simulink model "Robot"  (R2022b)
settings: Solver=FixedStepDiscrete  StartTime=0.0  StopTime=30  FixedStep=0.001  RelTol=1e-3
InitFcn:
  | load("BusConfig.mat");
undefined symbols (not defined in the file or in its folder): DiscIntNeverNeededParam
libraries: slrealtimeethercatlib x119, simulink x20
(part 1 of 7)
settings Model: SimulationMode=external  Creator=My-Dell-PC  LastModifiedBy=Lenovo
settings SolverCC: ConcurrentTasks=on  PositivePriorityOrder=on
settings OptimizationCC: BlockReduction=off  OptimizeBlockIOStorage=off
settings DebuggingCC: TasksWithSamePriorityMsg=none
settings HardwareCC: ProdBitPerLong=64  ProdLongLongMode=on  ProdHWDeviceType=Intel->x86-64 (Linux 64)
settings ModelReferenceCC: ModelReferenceNumInstancesAllowed=Single
settings RTWCC: Description=Simulink Real-Time  SystemTargetFile=slrealtime.tlc  TemplateMakefile=slrealtime_default_tmf  Toolchain=Simulink Real-Time Toolchain  BuildConfiguration=Faster Runs  CodeExecutionProfiling=on  TargetLang=C++
settings CodeAppCC: MaxIdLength=62

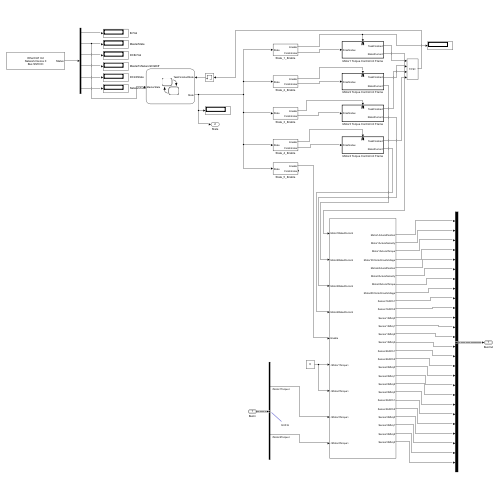
[thumbnail: Simulink's stored preview of the top-level diagram]
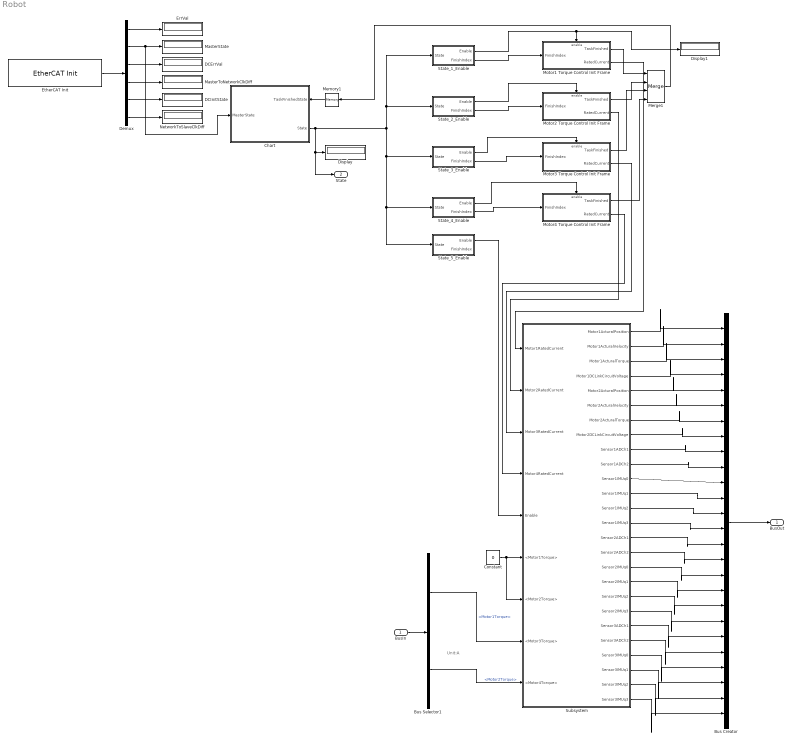
== system Robot ==
  note: Unit:A
  BusIn : Inport  OutDataTypeStr=Bus: ControlBus  BusOutputAsStruct=on
  Bus Creator : BusCreator  Inputs=26  OutDataTypeStr=Bus: SensingBus  NonVirtualBus=on
  Bus Selector1 : BusSelector  OutputSignals=Motor1Torque,Motor2Torque
  Chart : Stateflow chart  TreatAsAtomicUnit=on
      settings: PortSchema="{\"entries\":[{\"content\":{\"sides\":[{\"content\":{\"connectorIds\":[\"In2\"]},\"type\":\"ConnectorPlacement.EquallySpacedRectSide\",\"uuid\":\"7b8c9a1c-e183-4267-9de8-fd35f280369e\"},{\"content\":{\"connectorIds\":[\"In1\",\"Out1\"],\"side\":\"RIGHT\"},\"type\":\"ConnectorPlacement.EquallySpacedRectSide\",\"uuid\":\"78ba3a26-fd01-47d1-83ec-a88a58443a5d\"},{\"content\":{\"connectorIds\":[],\"side\":\"TOP\"},\"type\":\"ConnectorPlacement.EquallySpacedRectSide\",\"uuid\":\"d4867a2f-46dd-4a62-ab42-9e8e97143c91\"}]},\"type\":\"ConnectorPlacement.EquallySpacedConnector\",\"uuid\":\"fb86ace7-67ae-423a-b56c-83b1d93efbca\"}],\"packageUris\":[\"http://schema.mathworks.com/mf0/Connector/R2020b\"],\"version\":\"1.0\"}"
  Constant : Constant  Value=0
  "DCErrVal " : Display
  "DCInitState " : Display
  Demux : Demux  Outputs=6
  Display : Display
  Display1 : Display
  "ErrVal " : Display
  EtherCAT Init : slrealtimeethercatlib/EtherCAT Init  Priority=0  config_file=C:\Users\Lenovo\Desktop\Test03\FourMotorThreeSTMDevices.xml  device_id=0  pci_bus=0  pci_slot=0  pci_function=0  portnum=1  initstate=2  dctuning=0  enaDebug=1  enaDC=on  errLink=off  masterDbg=off  stateChgDbg=off  baseClock=off  masterCfg=off  logFile='c:\dbglog.txt'  sample_time=0.001000  DCMode=1
  "MasterState " : Display
  "MasterToNetworkClkDiff " : Display
  Memory1 : Memory
  Merge1 : Merge  Inputs=4
  Motor1 Torque Control Init Frame : Subsystem
  Motor2 Torque Control Init Frame : Subsystem
  Motor3 Torque Control Init Frame : Subsystem
  Motor4 Torque Control Init Frame : Subsystem
  "NetworkToSlaveClkDiff " : Display
  State_1_Enable : Subsystem  mask{TaskIndex=1}
  State_2_Enable : Subsystem  mask{TaskIndex=2}
  State_3_Enable : Subsystem  mask{TaskIndex=3}
  State_4_Enable : Subsystem  mask{TaskIndex=4}
  State_5_Enable : Subsystem  mask{TaskIndex=5}
  Subsystem : Subsystem
  BusOut : Outport  OutDataTypeStr=Bus: SensingBus  BusOutputAsStruct=on
  State : Outport  Port=2
  wires:
  Memory1/1 -> Chart/1(TaskFinishedState)
  State_1_Enable/2(FinishIndex) -> Motor1 Torque Control Init Frame/1(FinishIndex)
  Demux/1 -> "ErrVal "/1
  Merge1/1 -> Memory1/1
  Demux/6 -> "NetworkToSlaveClkDiff "/1
  Motor2 Torque Control Init Frame/1(TaskFinished) -> Merge1/2
  State_2_Enable/2(FinishIndex) -> Motor2 Torque Control Init Frame/1(FinishIndex)
  BusIn/1 -> Bus Selector1/1
  Motor1 Torque Control Init Frame/1(TaskFinished) -> Merge1/1
  Demux/4 -> "MasterToNetworkClkDiff "/1
  State_1_Enable/1(Enable) -> Motor1 Torque Control Init Frame/Enable, Display1/1
  State_2_Enable/1(Enable) -> Motor2 Torque Control Init Frame/Enable
  Demux/5 -> "DCInitState "/1
  EtherCAT Init/1 -> Demux/1
  Demux/2 -> "MasterState "/1, Chart/2(MasterState)
  Demux/3 -> "DCErrVal "/1
  Motor1 Torque Control Init Frame/2(RatedCurrent) -> Subsystem/1(Motor1RatedCurrent)
  Motor2 Torque Control Init Frame/2(RatedCurrent) -> Subsystem/2(Motor2RatedCurrent)
  State_5_Enable/1(Enable) -> Subsystem/5(Enable)
  Bus Selector1/1 -> Subsystem/8(<Motor3Torque>)  "<Motor1Torque>"
  Bus Selector1/2 -> Subsystem/9(<Motor4Torque>)  "<Motor2Torque>"
  Subsystem/1(Motor1ActuralPosition) -> Bus Creator/1
  Subsystem/2(Motor1ActuralVelocity) -> Bus Creator/2
  Subsystem/3(Motor1ActuralTorque) -> Bus Creator/3
  Subsystem/4(Motor1DCLinkCircuitVoltage) -> Bus Creator/4
  Subsystem/5(Motor2ActuralPosition) -> Bus Creator/5
  Subsystem/6(Motor2ActuralVelocity) -> Bus Creator/6
  Subsystem/7(Motor2ActuralTorque) -> Bus Creator/7
  Subsystem/8(Motor2DCLinkCircuitVoltage) -> Bus Creator/8
  Subsystem/9(Sensor1ADCh1) -> Bus Creator/9
  Subsystem/10(Sensor1ADCh2) -> Bus Creator/10
  Subsystem/11(Sensor1IMUq0) -> Bus Creator/11
  Subsystem/12(Sensor1IMUq1) -> Bus Creator/12
  Subsystem/13(Sensor1IMUq2) -> Bus Creator/13
  Subsystem/14(Sensor1IMUq3) -> Bus Creator/14
  Subsystem/15(Sensor2ADCh1) -> Bus Creator/15
  Subsystem/16(Sensor2ADCh2) -> Bus Creator/16
  Subsystem/17(Sensor2IMUq0) -> Bus Creator/17
  Subsystem/18(Sensor2IMUq1) -> Bus Creator/18
  Subsystem/19(Sensor2IMUq2) -> Bus Creator/19
  Subsystem/20(Sensor2IMUq3) -> Bus Creator/20
  Subsystem/21(Sensor3ADCh1) -> Bus Creator/21
  Subsystem/22(Sensor3ADCh2) -> Bus Creator/22
  Subsystem/23(Sensor3IMUq0) -> Bus Creator/23
  Subsystem/24(Sensor3IMUq1) -> Bus Creator/24
  Subsystem/25(Sensor3IMUq2) -> Bus Creator/25
  Subsystem/26(Sensor3IMUq3) -> Bus Creator/26
  Bus Creator/1 -> BusOut/1
  State_3_Enable/1(Enable) -> Motor3 Torque Control Init Frame/Enable
  State_3_Enable/2(FinishIndex) -> Motor3 Torque Control Init Frame/1(FinishIndex)
  Motor3 Torque Control Init Frame/1(TaskFinished) -> Merge1/3
  State_4_Enable/1(Enable) -> Motor4 Torque Control Init Frame/Enable
  State_4_Enable/2(FinishIndex) -> Motor4 Torque Control Init Frame/1(FinishIndex)
  Motor4 Torque Control Init Frame/1(TaskFinished) -> Merge1/4
  Motor3 Torque Control Init Frame/2(RatedCurrent) -> Subsystem/3(Motor3RatedCurrent)
  Motor4 Torque Control Init Frame/2(RatedCurrent) -> Subsystem/4(Motor4RatedCurrent)
  Constant/1 -> Subsystem/7(<Motor2Torque>), Subsystem/6(<Motor1Torque>)
  Chart/1(State) -> State_1_Enable/1(State), State_2_Enable/1(State), State_3_Enable/1(State), State_4_Enable/1(State), State_5_Enable/1(State), State/1, Display/1

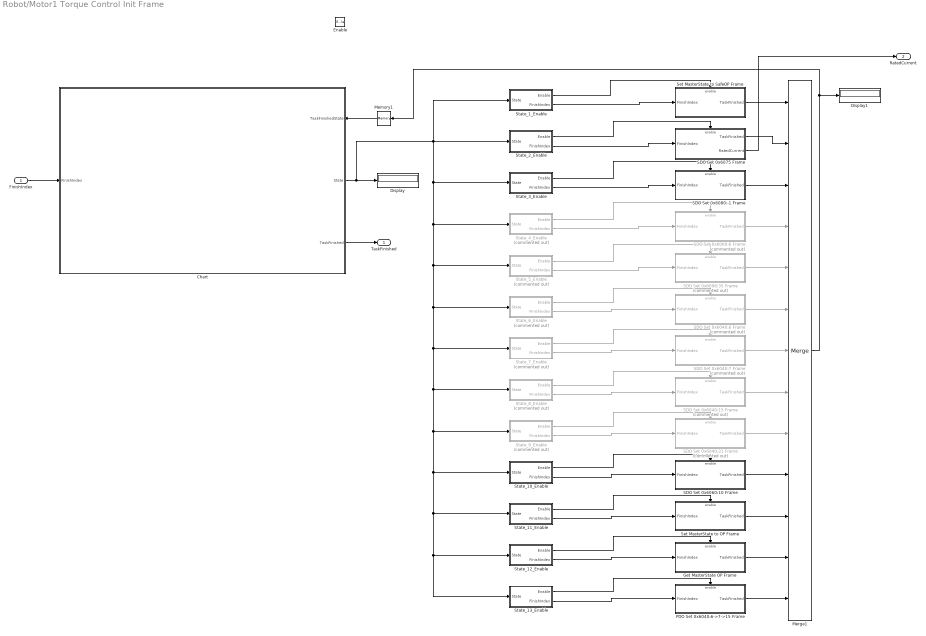
== system Robot/Motor1 Torque Control Init Frame ==
  FinishIndex : Inport
  Enable : EnablePort
  Chart : Stateflow chart  TreatAsAtomicUnit=on
      settings: PortSchema="{\"entries\":[{\"content\":{\"sides\":[{\"content\":{\"connectorIds\":[\"In1\"]},\"type\":\"ConnectorPlacement.EquallySpacedRectSide\",\"uuid\":\"58410e45-faf7-47e6-8ab9-12c4fba7eef9\"},{\"content\":{\"connectorIds\":[\"In2\",\"Out1\",\"Out2\"],\"side\":\"RIGHT\"},\"type\":\"ConnectorPlacement.EquallySpacedRectSide\",\"uuid\":\"b03d764f-4843-4a3f-88c0-0810c02290b2\"},{\"content\":{\"connectorIds\":[],\"side\":\"TOP\"},\"type\":\"ConnectorPlacement.EquallySpacedRectSide\",\"uuid\":\"d94600f9-94c4-4729-93e4-f24bdd83e939\"}]},\"type\":\"ConnectorPlacement.EquallySpacedConnector\",\"uuid\":\"f092a652-dcaf-4841-a284-968789b15227\"}],\"packageUris\":[\"http://schema.mathworks.com/mf0/Connector/R2020b\"],\"version\":\"1.0\"}"
  Display : Display
  Display1 : Display
  Get MasterState OP Frame : Subsystem
  Memory1 : Memory
  Merge1 : Merge  Inputs=13
  PDO Set 0x6040:6->7->15 Frame : Subsystem
  SDO Get 0x6075 Frame : Subsystem
  SDO Set 0x6040:15 Frame : Subsystem  Commented=on
  SDO Set 0x6040:31 Frame : Subsystem  Commented=on
  SDO Set 0x6040:6 Frame : Subsystem  Commented=on
  SDO Set 0x6040:7 Frame : Subsystem  Commented=on
  SDO Set 0x6060:10 Frame : Subsystem
  SDO Set 0x6060:6 Frame : Subsystem  Commented=on
  SDO Set 0x6080:-1 Frame : Subsystem
  SDO Set 0x6098:35 Frame : Subsystem  Commented=on
  Set MasterState to OP Frame : Subsystem
  Set MasterState to SafeOP Frame : Subsystem
  State_10_Enable : Subsystem  mask{TaskIndex=10}
  State_11_Enable : Subsystem  mask{TaskIndex=11}
  State_12_Enable : Subsystem  mask{TaskIndex=12}
  State_13_Enable : Subsystem  mask{TaskIndex=13}
  State_1_Enable : Subsystem  mask{TaskIndex=1}
  State_2_Enable : Subsystem  mask{TaskIndex=2}
  State_3_Enable : Subsystem  mask{TaskIndex=3}
  State_4_Enable : Subsystem  Commented=on  mask{TaskIndex=4}
  State_5_Enable : Subsystem  Commented=on  mask{TaskIndex=5}
  State_6_Enable : Subsystem  Commented=on  mask{TaskIndex=6}
  State_7_Enable : Subsystem  Commented=on  mask{TaskIndex=7}
  State_8_Enable : Subsystem  Commented=on  mask{TaskIndex=8}
  State_9_Enable : Subsystem  Commented=on  mask{TaskIndex=9}
  TaskFinished : Outport
  RatedCurrent : Outport  Port=2
  wires:
  SDO Get 0x6075 Frame/2(RatedCurrent) -> RatedCurrent/1
  Chart/1(State) -> State_1_Enable/1(State), State_2_Enable/1(State), State_3_Enable/1(State), State_4_Enable/1(State), State_5_Enable/1(State), State_6_Enable/1(State), State_7_Enable/1(State), State_8_Enable/1(State), State_9_Enable/1(State), State_10_Enable/1(State), State_11_Enable/1(State), State_13_Enable/1(State), State_12_Enable/1(State), Display/1
  Set MasterState to SafeOP Frame/1(TaskFinished) -> Merge1/1
  State_1_Enable/1(Enable) -> Set MasterState to SafeOP Frame/Enable
  State_1_Enable/2(FinishIndex) -> Set MasterState to SafeOP Frame/1(FinishIndex)
  State_2_Enable/1(Enable) -> SDO Get 0x6075 Frame/Enable
  State_2_Enable/2(FinishIndex) -> SDO Get 0x6075 Frame/1(FinishIndex)
  State_3_Enable/1(Enable) -> SDO Set 0x6080:-1 Frame/Enable
  State_3_Enable/2(FinishIndex) -> SDO Set 0x6080:-1 Frame/1(FinishIndex)
  State_4_Enable/1(Enable) -> SDO Set 0x6060:6 Frame/Enable
  State_4_Enable/2(FinishIndex) -> SDO Set 0x6060:6 Frame/1(FinishIndex)
  State_5_Enable/1(Enable) -> SDO Set 0x6098:35 Frame/Enable
  State_5_Enable/2(FinishIndex) -> SDO Set 0x6098:35 Frame/1(FinishIndex)
  State_6_Enable/1(Enable) -> SDO Set 0x6040:6 Frame/Enable
  State_6_Enable/2(FinishIndex) -> SDO Set 0x6040:6 Frame/1(FinishIndex)
  State_7_Enable/1(Enable) -> SDO Set 0x6040:7 Frame/Enable
  State_7_Enable/2(FinishIndex) -> SDO Set 0x6040:7 Frame/1(FinishIndex)
  State_8_Enable/2(FinishIndex) -> SDO Set 0x6040:15 Frame/1(FinishIndex)
  State_8_Enable/1(Enable) -> SDO Set 0x6040:15 Frame/Enable
  State_9_Enable/1(Enable) -> SDO Set 0x6040:31 Frame/Enable
  State_9_Enable/2(FinishIndex) -> SDO Set 0x6040:31 Frame/1(FinishIndex)
  State_10_Enable/1(Enable) -> SDO Set 0x6060:10 Frame/Enable
  State_10_Enable/2(FinishIndex) -> SDO Set 0x6060:10 Frame/1(FinishIndex)
  State_11_Enable/1(Enable) -> Set MasterState to OP Frame/Enable
  State_11_Enable/2(FinishIndex) -> Set MasterState to OP Frame/1(FinishIndex)
  State_12_Enable/1(Enable) -> Get MasterState OP Frame/Enable
  State_12_Enable/2(FinishIndex) -> Get MasterState OP Frame/1(FinishIndex)
  State_13_Enable/1(Enable) -> PDO Set 0x6040:6->7->15 Frame/Enable
  State_13_Enable/2(FinishIndex) -> PDO Set 0x6040:6->7->15 Frame/1(FinishIndex)
  SDO Get 0x6075 Frame/1(TaskFinished) -> Merge1/2
  SDO Set 0x6080:-1 Frame/1(TaskFinished) -> Merge1/3
  SDO Set 0x6060:6 Frame/1(TaskFinished) -> Merge1/4
  SDO Set 0x6098:35 Frame/1(TaskFinished) -> Merge1/5
  SDO Set 0x6040:6 Frame/1(TaskFinished) -> Merge1/6
  SDO Set 0x6040:7 Frame/1(TaskFinished) -> Merge1/7
  SDO Set 0x6040:15 Frame/1(TaskFinished) -> Merge1/8
  SDO Set 0x6040:31 Frame/1(TaskFinished) -> Merge1/9
  SDO Set 0x6060:10 Frame/1(TaskFinished) -> Merge1/10
  Set MasterState to OP Frame/1(TaskFinished) -> Merge1/11
  Get MasterState OP Frame/1(TaskFinished) -> Merge1/12
  PDO Set 0x6040:6->7->15 Frame/1(TaskFinished) -> Merge1/13
  Merge1/1 -> Display1/1, Memory1/1
  Chart/2(TaskFinished) -> TaskFinished/1
  FinishIndex/1 -> Chart/1(FinishIndex)
  Memory1/1 -> Chart/2(TaskFinishedState)

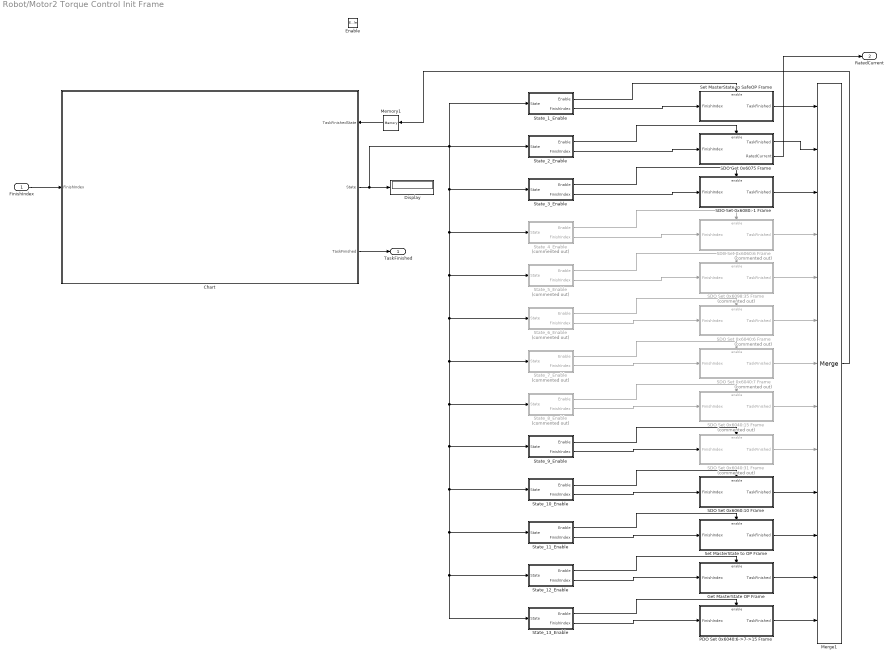
== system Robot/Motor2 Torque Control Init Frame ==
  FinishIndex : Inport
  Enable : EnablePort
  Chart : Stateflow chart  TreatAsAtomicUnit=on
      settings: PortSchema="{\"entries\":[{\"content\":{\"sides\":[{\"content\":{\"connectorIds\":[\"In1\"]},\"type\":\"ConnectorPlacement.EquallySpacedRectSide\",\"uuid\":\"58410e45-faf7-47e6-8ab9-12c4fba7eef9\"},{\"content\":{\"connectorIds\":[\"In2\",\"Out1\",\"Out2\"],\"side\":\"RIGHT\"},\"type\":\"ConnectorPlacement.EquallySpacedRectSide\",\"uuid\":\"b03d764f-4843-4a3f-88c0-0810c02290b2\"},{\"content\":{\"connectorIds\":[],\"side\":\"TOP\"},\"type\":\"ConnectorPlacement.EquallySpacedRectSide\",\"uuid\":\"d94600f9-94c4-4729-93e4-f24bdd83e939\"}]},\"type\":\"ConnectorPlacement.EquallySpacedConnector\",\"uuid\":\"f092a652-dcaf-4841-a284-968789b15227\"}],\"packageUris\":[\"http://schema.mathworks.com/mf0/Connector/R2020b\"],\"version\":\"1.0\"}"
  Display : Display
  Get MasterState OP Frame : Subsystem
  Memory1 : Memory
  Merge1 : Merge  Inputs=13
  PDO Set 0x6040:6->7->15 Frame : Subsystem
  SDO Get 0x6075 Frame : Subsystem
  SDO Set 0x6040:15 Frame : Subsystem  Commented=on
  SDO Set 0x6040:31 Frame : Subsystem  Commented=on
  SDO Set 0x6040:6 Frame : Subsystem  Commented=on
  SDO Set 0x6040:7 Frame : Subsystem  Commented=on
  SDO Set 0x6060:10 Frame : Subsystem
  SDO Set 0x6060:6 Frame : Subsystem  Commented=on
  SDO Set 0x6080:-1 Frame : Subsystem
  SDO Set 0x6098:35 Frame : Subsystem  Commented=on
  Set MasterState to OP Frame : Subsystem
  Set MasterState to SafeOP Frame : Subsystem
  State_10_Enable : Subsystem  mask{TaskIndex=10}
  State_11_Enable : Subsystem  mask{TaskIndex=11}
  State_12_Enable : Subsystem  mask{TaskIndex=12}
  State_13_Enable : Subsystem  mask{TaskIndex=13}
  State_1_Enable : Subsystem  mask{TaskIndex=1}
  State_2_Enable : Subsystem  mask{TaskIndex=2}
  State_3_Enable : Subsystem  mask{TaskIndex=3}
  State_4_Enable : Subsystem  Commented=on  mask{TaskIndex=4}
  State_5_Enable : Subsystem  Commented=on  mask{TaskIndex=5}
  State_6_Enable : Subsystem  Commented=on  mask{TaskIndex=6}
  State_7_Enable : Subsystem  Commented=on  mask{TaskIndex=7}
  State_8_Enable : Subsystem  Commented=on  mask{TaskIndex=8}
  State_9_Enable : Subsystem  mask{TaskIndex=9}
  TaskFinished : Outport
  RatedCurrent : Outport  Port=2
  wires:
  SDO Get 0x6075 Frame/2(RatedCurrent) -> RatedCurrent/1
  Chart/1(State) -> State_1_Enable/1(State), State_2_Enable/1(State), State_3_Enable/1(State), State_4_Enable/1(State), State_5_Enable/1(State), State_6_Enable/1(State), State_7_Enable/1(State), State_8_Enable/1(State), State_9_Enable/1(State), State_10_Enable/1(State), State_11_Enable/1(State), State_13_Enable/1(State), State_12_Enable/1(State), Display/1
  Set MasterState to SafeOP Frame/1(TaskFinished) -> Merge1/1
  State_1_Enable/1(Enable) -> Set MasterState to SafeOP Frame/Enable
  State_1_Enable/2(FinishIndex) -> Set MasterState to SafeOP Frame/1(FinishIndex)
  State_2_Enable/1(Enable) -> SDO Get 0x6075 Frame/Enable
  State_2_Enable/2(FinishIndex) -> SDO Get 0x6075 Frame/1(FinishIndex)
  State_3_Enable/1(Enable) -> SDO Set 0x6080:-1 Frame/Enable
  State_3_Enable/2(FinishIndex) -> SDO Set 0x6080:-1 Frame/1(FinishIndex)
  State_4_Enable/1(Enable) -> SDO Set 0x6060:6 Frame/Enable
  State_4_Enable/2(FinishIndex) -> SDO Set 0x6060:6 Frame/1(FinishIndex)
  State_5_Enable/1(Enable) -> SDO Set 0x6098:35 Frame/Enable
  State_5_Enable/2(FinishIndex) -> SDO Set 0x6098:35 Frame/1(FinishIndex)
  State_6_Enable/1(Enable) -> SDO Set 0x6040:6 Frame/Enable
  State_6_Enable/2(FinishIndex) -> SDO Set 0x6040:6 Frame/1(FinishIndex)
  State_7_Enable/1(Enable) -> SDO Set 0x6040:7 Frame/Enable
  State_7_Enable/2(FinishIndex) -> SDO Set 0x6040:7 Frame/1(FinishIndex)
  State_8_Enable/2(FinishIndex) -> SDO Set 0x6040:15 Frame/1(FinishIndex)
  State_8_Enable/1(Enable) -> SDO Set 0x6040:15 Frame/Enable
  State_9_Enable/1(Enable) -> SDO Set 0x6040:31 Frame/Enable
  State_9_Enable/2(FinishIndex) -> SDO Set 0x6040:31 Frame/1(FinishIndex)
  State_10_Enable/1(Enable) -> SDO Set 0x6060:10 Frame/Enable
  State_10_Enable/2(FinishIndex) -> SDO Set 0x6060:10 Frame/1(FinishIndex)
  State_11_Enable/1(Enable) -> Set MasterState to OP Frame/Enable
  State_11_Enable/2(FinishIndex) -> Set MasterState to OP Frame/1(FinishIndex)
  State_12_Enable/1(Enable) -> Get MasterState OP Frame/Enable
  State_12_Enable/2(FinishIndex) -> Get MasterState OP Frame/1(FinishIndex)
  State_13_Enable/1(Enable) -> PDO Set 0x6040:6->7->15 Frame/Enable
  State_13_Enable/2(FinishIndex) -> PDO Set 0x6040:6->7->15 Frame/1(FinishIndex)
  SDO Get 0x6075 Frame/1(TaskFinished) -> Merge1/2
  SDO Set 0x6080:-1 Frame/1(TaskFinished) -> Merge1/3
  SDO Set 0x6060:6 Frame/1(TaskFinished) -> Merge1/4
  SDO Set 0x6098:35 Frame/1(TaskFinished) -> Merge1/5
  SDO Set 0x6040:6 Frame/1(TaskFinished) -> Merge1/6
  SDO Set 0x6040:7 Frame/1(TaskFinished) -> Merge1/7
  SDO Set 0x6040:15 Frame/1(TaskFinished) -> Merge1/8
  SDO Set 0x6040:31 Frame/1(TaskFinished) -> Merge1/9
  SDO Set 0x6060:10 Frame/1(TaskFinished) -> Merge1/10
  Set MasterState to OP Frame/1(TaskFinished) -> Merge1/11
  Get MasterState OP Frame/1(TaskFinished) -> Merge1/12
  PDO Set 0x6040:6->7->15 Frame/1(TaskFinished) -> Merge1/13
  Merge1/1 -> Memory1/1
  Chart/2(TaskFinished) -> TaskFinished/1
  FinishIndex/1 -> Chart/1(FinishIndex)
  Memory1/1 -> Chart/2(TaskFinishedState)

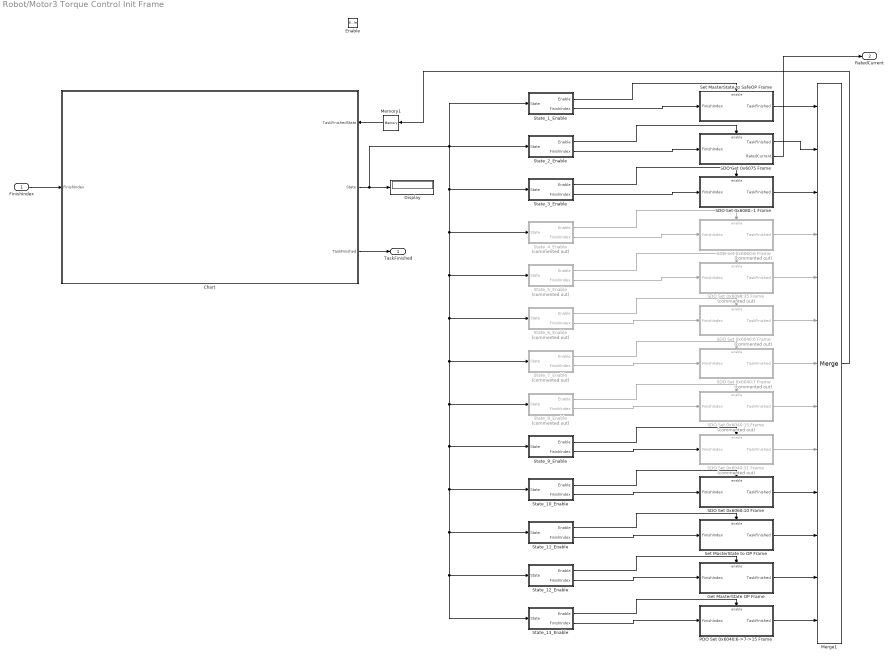
== system Robot/Motor3 Torque Control Init Frame ==
  FinishIndex : Inport
  Enable : EnablePort
  Chart : Stateflow chart  TreatAsAtomicUnit=on
      settings: PortSchema="{\"entries\":[{\"content\":{\"sides\":[{\"content\":{\"connectorIds\":[\"In1\"]},\"type\":\"ConnectorPlacement.EquallySpacedRectSide\",\"uuid\":\"58410e45-faf7-47e6-8ab9-12c4fba7eef9\"},{\"content\":{\"connectorIds\":[\"In2\",\"Out1\",\"Out2\"],\"side\":\"RIGHT\"},\"type\":\"ConnectorPlacement.EquallySpacedRectSide\",\"uuid\":\"b03d764f-4843-4a3f-88c0-0810c02290b2\"},{\"content\":{\"connectorIds\":[],\"side\":\"TOP\"},\"type\":\"ConnectorPlacement.EquallySpacedRectSide\",\"uuid\":\"d94600f9-94c4-4729-93e4-f24bdd83e939\"}]},\"type\":\"ConnectorPlacement.EquallySpacedConnector\",\"uuid\":\"f092a652-dcaf-4841-a284-968789b15227\"}],\"packageUris\":[\"http://schema.mathworks.com/mf0/Connector/R2020b\"],\"version\":\"1.0\"}"
  Display : Display
  Get MasterState OP Frame : Subsystem
  Memory1 : Memory
  Merge1 : Merge  Inputs=13
  PDO Set 0x6040:6->7->15 Frame : Subsystem
  SDO Get 0x6075 Frame : Subsystem
  SDO Set 0x6040:15 Frame : Subsystem  Commented=on
  SDO Set 0x6040:31 Frame : Subsystem  Commented=on
  SDO Set 0x6040:6 Frame : Subsystem  Commented=on
  SDO Set 0x6040:7 Frame : Subsystem  Commented=on
  SDO Set 0x6060:10 Frame : Subsystem
  SDO Set 0x6060:6 Frame : Subsystem  Commented=on
  SDO Set 0x6080:-1 Frame : Subsystem
  SDO Set 0x6098:35 Frame : Subsystem  Commented=on
  Set MasterState to OP Frame : Subsystem
  Set MasterState to SafeOP Frame : Subsystem
  State_10_Enable : Subsystem  mask{TaskIndex=10}
  State_11_Enable : Subsystem  mask{TaskIndex=11}
  State_12_Enable : Subsystem  mask{TaskIndex=12}
  State_13_Enable : Subsystem  mask{TaskIndex=13}
  State_1_Enable : Subsystem  mask{TaskIndex=1}
  State_2_Enable : Subsystem  mask{TaskIndex=2}
  State_3_Enable : Subsystem  mask{TaskIndex=3}
  State_4_Enable : Subsystem  Commented=on  mask{TaskIndex=4}
  State_5_Enable : Subsystem  Commented=on  mask{TaskIndex=5}
  State_6_Enable : Subsystem  Commented=on  mask{TaskIndex=6}
  State_7_Enable : Subsystem  Commented=on  mask{TaskIndex=7}
  State_8_Enable : Subsystem  Commented=on  mask{TaskIndex=8}
  State_9_Enable : Subsystem  mask{TaskIndex=9}
  TaskFinished : Outport
  RatedCurrent : Outport  Port=2
  wires:
  SDO Get 0x6075 Frame/2(RatedCurrent) -> RatedCurrent/1
  Chart/1(State) -> State_1_Enable/1(State), State_2_Enable/1(State), State_3_Enable/1(State), State_4_Enable/1(State), State_5_Enable/1(State), State_6_Enable/1(State), State_7_Enable/1(State), State_8_Enable/1(State), State_9_Enable/1(State), State_10_Enable/1(State), State_11_Enable/1(State), State_13_Enable/1(State), State_12_Enable/1(State), Display/1
  Set MasterState to SafeOP Frame/1(TaskFinished) -> Merge1/1
  State_1_Enable/1(Enable) -> Set MasterState to SafeOP Frame/Enable
  State_1_Enable/2(FinishIndex) -> Set MasterState to SafeOP Frame/1(FinishIndex)
  State_2_Enable/1(Enable) -> SDO Get 0x6075 Frame/Enable
  State_2_Enable/2(FinishIndex) -> SDO Get 0x6075 Frame/1(FinishIndex)
  State_3_Enable/1(Enable) -> SDO Set 0x6080:-1 Frame/Enable
  State_3_Enable/2(FinishIndex) -> SDO Set 0x6080:-1 Frame/1(FinishIndex)
  State_4_Enable/1(Enable) -> SDO Set 0x6060:6 Frame/Enable
  State_4_Enable/2(FinishIndex) -> SDO Set 0x6060:6 Frame/1(FinishIndex)
  State_5_Enable/1(Enable) -> SDO Set 0x6098:35 Frame/Enable
  State_5_Enable/2(FinishIndex) -> SDO Set 0x6098:35 Frame/1(FinishIndex)
  State_6_Enable/1(Enable) -> SDO Set 0x6040:6 Frame/Enable
  State_6_Enable/2(FinishIndex) -> SDO Set 0x6040:6 Frame/1(FinishIndex)
  State_7_Enable/1(Enable) -> SDO Set 0x6040:7 Frame/Enable
  State_7_Enable/2(FinishIndex) -> SDO Set 0x6040:7 Frame/1(FinishIndex)
  State_8_Enable/2(FinishIndex) -> SDO Set 0x6040:15 Frame/1(FinishIndex)
  State_8_Enable/1(Enable) -> SDO Set 0x6040:15 Frame/Enable
  State_9_Enable/1(Enable) -> SDO Set 0x6040:31 Frame/Enable
  State_9_Enable/2(FinishIndex) -> SDO Set 0x6040:31 Frame/1(FinishIndex)
  State_10_Enable/1(Enable) -> SDO Set 0x6060:10 Frame/Enable
  State_10_Enable/2(FinishIndex) -> SDO Set 0x6060:10 Frame/1(FinishIndex)
  State_11_Enable/1(Enable) -> Set MasterState to OP Frame/Enable
  State_11_Enable/2(FinishIndex) -> Set MasterState to OP Frame/1(FinishIndex)
  State_12_Enable/1(Enable) -> Get MasterState OP Frame/Enable
  State_12_Enable/2(FinishIndex) -> Get MasterState OP Frame/1(FinishIndex)
  State_13_Enable/1(Enable) -> PDO Set 0x6040:6->7->15 Frame/Enable
  State_13_Enable/2(FinishIndex) -> PDO Set 0x6040:6->7->15 Frame/1(FinishIndex)
  SDO Get 0x6075 Frame/1(TaskFinished) -> Merge1/2
  SDO Set 0x6080:-1 Frame/1(TaskFinished) -> Merge1/3
  SDO Set 0x6060:6 Frame/1(TaskFinished) -> Merge1/4
  SDO Set 0x6098:35 Frame/1(TaskFinished) -> Merge1/5
  SDO Set 0x6040:6 Frame/1(TaskFinished) -> Merge1/6
  SDO Set 0x6040:7 Frame/1(TaskFinished) -> Merge1/7
  SDO Set 0x6040:15 Frame/1(TaskFinished) -> Merge1/8
  SDO Set 0x6040:31 Frame/1(TaskFinished) -> Merge1/9
  SDO Set 0x6060:10 Frame/1(TaskFinished) -> Merge1/10
  Set MasterState to OP Frame/1(TaskFinished) -> Merge1/11
  Get MasterState OP Frame/1(TaskFinished) -> Merge1/12
  PDO Set 0x6040:6->7->15 Frame/1(TaskFinished) -> Merge1/13
  Merge1/1 -> Memory1/1
  Chart/2(TaskFinished) -> TaskFinished/1
  FinishIndex/1 -> Chart/1(FinishIndex)
  Memory1/1 -> Chart/2(TaskFinishedState)

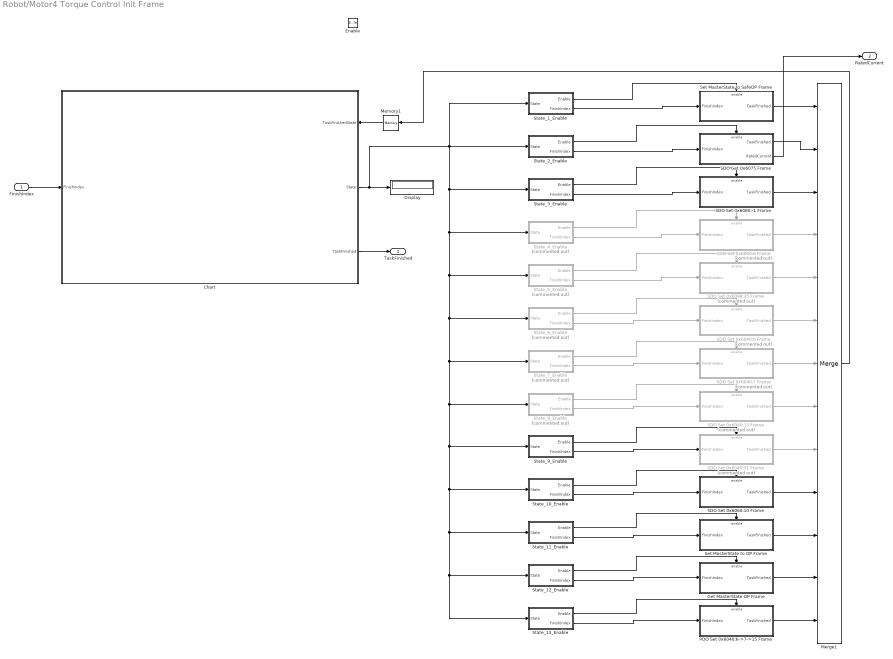
== system Robot/Motor4 Torque Control Init Frame ==
  FinishIndex : Inport
  Enable : EnablePort
  Chart : Stateflow chart  TreatAsAtomicUnit=on
      settings: PortSchema="{\"entries\":[{\"content\":{\"sides\":[{\"content\":{\"connectorIds\":[\"In1\"]},\"type\":\"ConnectorPlacement.EquallySpacedRectSide\",\"uuid\":\"58410e45-faf7-47e6-8ab9-12c4fba7eef9\"},{\"content\":{\"connectorIds\":[\"In2\",\"Out1\",\"Out2\"],\"side\":\"RIGHT\"},\"type\":\"ConnectorPlacement.EquallySpacedRectSide\",\"uuid\":\"b03d764f-4843-4a3f-88c0-0810c02290b2\"},{\"content\":{\"connectorIds\":[],\"side\":\"TOP\"},\"type\":\"ConnectorPlacement.EquallySpacedRectSide\",\"uuid\":\"d94600f9-94c4-4729-93e4-f24bdd83e939\"}]},\"type\":\"ConnectorPlacement.EquallySpacedConnector\",\"uuid\":\"f092a652-dcaf-4841-a284-968789b15227\"}],\"packageUris\":[\"http://schema.mathworks.com/mf0/Connector/R2020b\"],\"version\":\"1.0\"}"
  Display : Display
  Get MasterState OP Frame : Subsystem
  Memory1 : Memory
  Merge1 : Merge  Inputs=13
  PDO Set 0x6040:6->7->15 Frame : Subsystem
  SDO Get 0x6075 Frame : Subsystem
  SDO Set 0x6040:15 Frame : Subsystem  Commented=on
  SDO Set 0x6040:31 Frame : Subsystem  Commented=on
  SDO Set 0x6040:6 Frame : Subsystem  Commented=on
  SDO Set 0x6040:7 Frame : Subsystem  Commented=on
  SDO Set 0x6060:10 Frame : Subsystem
  SDO Set 0x6060:6 Frame : Subsystem  Commented=on
  SDO Set 0x6080:-1 Frame : Subsystem
  SDO Set 0x6098:35 Frame : Subsystem  Commented=on
  Set MasterState to OP Frame : Subsystem
  Set MasterState to SafeOP Frame : Subsystem
  State_10_Enable : Subsystem  mask{TaskIndex=10}
  State_11_Enable : Subsystem  mask{TaskIndex=11}
  State_12_Enable : Subsystem  mask{TaskIndex=12}
  State_13_Enable : Subsystem  mask{TaskIndex=13}
  State_1_Enable : Subsystem  mask{TaskIndex=1}
  State_2_Enable : Subsystem  mask{TaskIndex=2}
  State_3_Enable : Subsystem  mask{TaskIndex=3}
  State_4_Enable : Subsystem  Commented=on  mask{TaskIndex=4}
  State_5_Enable : Subsystem  Commented=on  mask{TaskIndex=5}
  State_6_Enable : Subsystem  Commented=on  mask{TaskIndex=6}
  State_7_Enable : Subsystem  Commented=on  mask{TaskIndex=7}
  State_8_Enable : Subsystem  Commented=on  mask{TaskIndex=8}
  State_9_Enable : Subsystem  mask{TaskIndex=9}
  TaskFinished : Outport
  RatedCurrent : Outport  Port=2
  wires:
  SDO Get 0x6075 Frame/2(RatedCurrent) -> RatedCurrent/1
  Chart/1(State) -> State_1_Enable/1(State), State_2_Enable/1(State), State_3_Enable/1(State), State_4_Enable/1(State), State_5_Enable/1(State), State_6_Enable/1(State), State_7_Enable/1(State), State_8_Enable/1(State), State_9_Enable/1(State), State_10_Enable/1(State), State_11_Enable/1(State), State_13_Enable/1(State), State_12_Enable/1(State), Display/1
  Set MasterState to SafeOP Frame/1(TaskFinished) -> Merge1/1
  State_1_Enable/1(Enable) -> Set MasterState to SafeOP Frame/Enable
  State_1_Enable/2(FinishIndex) -> Set MasterState to SafeOP Frame/1(FinishIndex)
  State_2_Enable/1(Enable) -> SDO Get 0x6075 Frame/Enable
  State_2_Enable/2(FinishIndex) -> SDO Get 0x6075 Frame/1(FinishIndex)
  State_3_Enable/1(Enable) -> SDO Set 0x6080:-1 Frame/Enable
  State_3_Enable/2(FinishIndex) -> SDO Set 0x6080:-1 Frame/1(FinishIndex)
  State_4_Enable/1(Enable) -> SDO Set 0x6060:6 Frame/Enable
  State_4_Enable/2(FinishIndex) -> SDO Set 0x6060:6 Frame/1(FinishIndex)
  State_5_Enable/1(Enable) -> SDO Set 0x6098:35 Frame/Enable
  State_5_Enable/2(FinishIndex) -> SDO Set 0x6098:35 Frame/1(FinishIndex)
  State_6_Enable/1(Enable) -> SDO Set 0x6040:6 Frame/Enable
  State_6_Enable/2(FinishIndex) -> SDO Set 0x6040:6 Frame/1(FinishIndex)
  State_7_Enable/1(Enable) -> SDO Set 0x6040:7 Frame/Enable
  State_7_Enable/2(FinishIndex) -> SDO Set 0x6040:7 Frame/1(FinishIndex)
  State_8_Enable/2(FinishIndex) -> SDO Set 0x6040:15 Frame/1(FinishIndex)
  State_8_Enable/1(Enable) -> SDO Set 0x6040:15 Frame/Enable
  State_9_Enable/1(Enable) -> SDO Set 0x6040:31 Frame/Enable
  State_9_Enable/2(FinishIndex) -> SDO Set 0x6040:31 Frame/1(FinishIndex)
  State_10_Enable/1(Enable) -> SDO Set 0x6060:10 Frame/Enable
  State_10_Enable/2(FinishIndex) -> SDO Set 0x6060:10 Frame/1(FinishIndex)
  State_11_Enable/1(Enable) -> Set MasterState to OP Frame/Enable
  State_11_Enable/2(FinishIndex) -> Set MasterState to OP Frame/1(FinishIndex)
  State_12_Enable/1(Enable) -> Get MasterState OP Frame/Enable
  State_12_Enable/2(FinishIndex) -> Get MasterState OP Frame/1(FinishIndex)
  State_13_Enable/1(Enable) -> PDO Set 0x6040:6->7->15 Frame/Enable
  State_13_Enable/2(FinishIndex) -> PDO Set 0x6040:6->7->15 Frame/1(FinishIndex)
  SDO Get 0x6075 Frame/1(TaskFinished) -> Merge1/2
  SDO Set 0x6080:-1 Frame/1(TaskFinished) -> Merge1/3
  SDO Set 0x6060:6 Frame/1(TaskFinished) -> Merge1/4
  SDO Set 0x6098:35 Frame/1(TaskFinished) -> Merge1/5
  SDO Set 0x6040:6 Frame/1(TaskFinished) -> Merge1/6
  SDO Set 0x6040:7 Frame/1(TaskFinished) -> Merge1/7
  SDO Set 0x6040:15 Frame/1(TaskFinished) -> Merge1/8
  SDO Set 0x6040:31 Frame/1(TaskFinished) -> Merge1/9
  SDO Set 0x6060:10 Frame/1(TaskFinished) -> Merge1/10
  Set MasterState to OP Frame/1(TaskFinished) -> Merge1/11
  Get MasterState OP Frame/1(TaskFinished) -> Merge1/12
  PDO Set 0x6040:6->7->15 Frame/1(TaskFinished) -> Merge1/13
  Merge1/1 -> Memory1/1
  Chart/2(TaskFinished) -> TaskFinished/1
  FinishIndex/1 -> Chart/1(FinishIndex)
  Memory1/1 -> Chart/2(TaskFinishedState)

== system Robot/State_1_Enable ==
  State : Inport
  Subsystem : Subsystem
  Switch Case : SwitchCase  CaseConditions={TaskIndex}
  Enable : Outport
  FinishIndex : Outport  Port=2
  wires:
  Switch Case/2 -> Subsystem/2(Case Default)
  Switch Case/1 -> Subsystem/1(Case)
  Subsystem/2(FinishIndex) -> FinishIndex/1
  Subsystem/1(Enable) -> Enable/1
  State/1 -> Switch Case/1

== system Robot/State_2_Enable ==
  State : Inport
  Subsystem : Subsystem
  Switch Case : SwitchCase  CaseConditions={TaskIndex}
  Enable : Outport
  FinishIndex : Outport  Port=2
  wires:
  Switch Case/2 -> Subsystem/2(Case Default)
  Switch Case/1 -> Subsystem/1(Case)
  Subsystem/2(FinishIndex) -> FinishIndex/1
  Subsystem/1(Enable) -> Enable/1
  State/1 -> Switch Case/1

== system Robot/State_3_Enable ==
  State : Inport
  Subsystem : Subsystem
  Switch Case : SwitchCase  CaseConditions={TaskIndex}
  Enable : Outport
  FinishIndex : Outport  Port=2
  wires:
  Switch Case/2 -> Subsystem/2(Case Default)
  Switch Case/1 -> Subsystem/1(Case)
  Subsystem/2(FinishIndex) -> FinishIndex/1
  Subsystem/1(Enable) -> Enable/1
  State/1 -> Switch Case/1

== system Robot/State_4_Enable ==
  State : Inport
  Subsystem : Subsystem
  Switch Case : SwitchCase  CaseConditions={TaskIndex}
  Enable : Outport
  FinishIndex : Outport  Port=2
  wires:
  Switch Case/2 -> Subsystem/2(Case Default)
  Switch Case/1 -> Subsystem/1(Case)
  Subsystem/2(FinishIndex) -> FinishIndex/1
  Subsystem/1(Enable) -> Enable/1
  State/1 -> Switch Case/1

== system Robot/State_5_Enable ==
  State : Inport
  Subsystem : Subsystem
  Switch Case : SwitchCase  CaseConditions={TaskIndex}
  Enable : Outport
  FinishIndex : Outport  Port=2
  wires:
  Switch Case/2 -> Subsystem/2(Case Default)
  Switch Case/1 -> Subsystem/1(Case)
  Subsystem/2(FinishIndex) -> FinishIndex/1
  Subsystem/1(Enable) -> Enable/1
  State/1 -> Switch Case/1

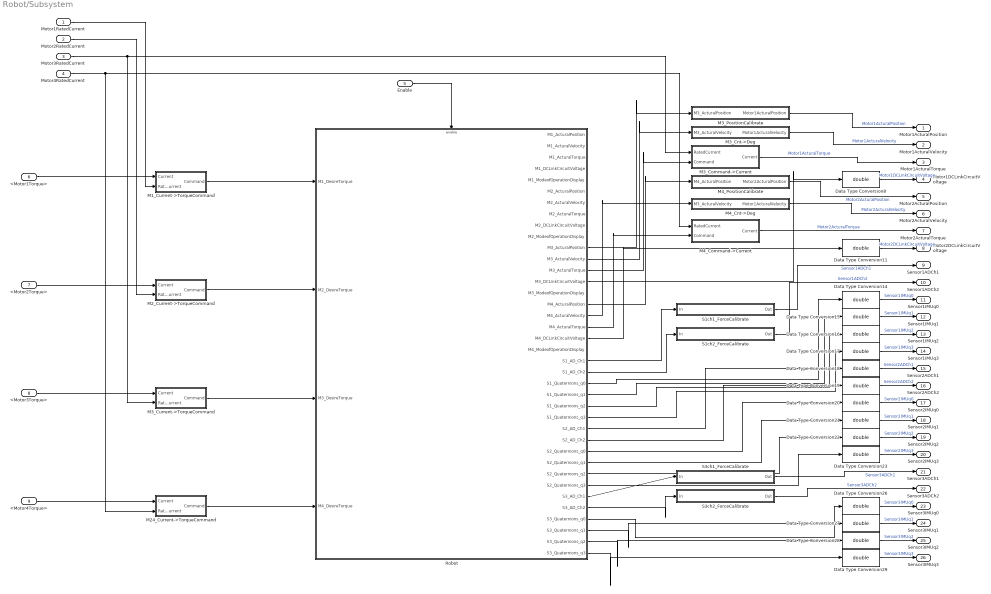
== system Robot/Subsystem ==
  Motor1RatedCurrent : Inport
  Motor2RatedCurrent : Inport  Port=2
  Motor3RatedCurrent : Inport  Port=3
  Motor4RatedCurrent : Inport  Port=4
  Enable : Inport  Port=5
  <Motor1Torque> : Inport  Port=6
  <Motor2Torque> : Inport  Port=7
  <Motor3Torque> : Inport  Port=8
  <Motor4Torque> : Inport  Port=9
  Data Type Conversion{8,11,14..23,26..29} (16 alike) : DataTypeConversion  OutDataTypeStr=double  SaturateOnIntegerOverflow=off  RndMeth=Floor
  M1_Current->TorqueCommand : Subsystem
  M24_Current->TorqueCommand : Subsystem
  M2_Current->TorqueCommand : Subsystem
  M3_Cnt->Deg : Subsystem
  M3_Command->Current : Subsystem
  M3_Current->TorqueCommand : Subsystem
  M3_PositionCalibrate : Subsystem
  M4_Cnt->Deg : Subsystem
  M4_Command->Current : Subsystem
  M4_PositionCalibrate : Subsystem
  Robot : Subsystem
  S1ch1_ForceCalibrate : Subsystem
  S1ch2_ForceCalibrate : Subsystem
  S3ch1_ForceCalibrate : Subsystem
  S3ch2_ForceCalibrate : Subsystem
  Motor1ActuralPosition : Outport
  Motor1ActuralVelocity : Outport  Port=2
  Motor1ActuralTorque : Outport  Port=3
  Motor1DCLinkCircuitVoltage : Outport  Port=4
  Motor2ActuralPosition : Outport  Port=5
  Motor2ActuralVelocity : Outport  Port=6
  Motor2ActuralTorque : Outport  Port=7
  Motor2DCLinkCircuitVoltage : Outport  Port=8
  Sensor1ADCh1 : Outport  Port=9
  Sensor1ADCh2 : Outport  Port=10
  Sensor1IMUq0 : Outport  Port=11
  Sensor1IMUq1 : Outport  Port=12
  Sensor1IMUq2 : Outport  Port=13
  Sensor1IMUq3 : Outport  Port=14
  Sensor2ADCh1 : Outport  Port=15
  Sensor2ADCh2 : Outport  Port=16
  Sensor2IMUq0 : Outport  Port=17
  Sensor2IMUq1 : Outport  Port=18
  Sensor2IMUq2 : Outport  Port=19
  Sensor2IMUq3 : Outport  Port=20
  Sensor3ADCh1 : Outport  Port=21
  Sensor3ADCh2 : Outport  Port=22
  Sensor3IMUq0 : Outport  Port=23
  Sensor3IMUq1 : Outport  Port=24
  Sensor3IMUq2 : Outport  Port=25
  Sensor3IMUq3 : Outport  Port=26
  wires:
  Data Type Conversion23/1 -> Sensor2IMUq3/1  "Sensor2IMUq3"
  Data Type Conversion11/1 -> Motor2DCLinkCircuitVoltage/1  "Motor2DCLinkCircuitVoltage"
  Robot/35(S3_Quaternions_q0) -> Data Type Conversion26/1
  Data Type Conversion26/1 -> Sensor3IMUq0/1  "Sensor3IMUq0"
  Robot/36(S3_Quaternions_q1) -> Data Type Conversion27/1
  Robot/27(S2_AD_Ch1) -> Data Type Conversion18/1
  M1_Current->TorqueCommand/1(Command) -> Robot/1(M1_DesireTorque)
  Data Type Conversion19/1 -> Sensor2ADCh2/1  "Sensor2ADCh2"
  Robot/24(S1_Quaternions_q1) -> Data Type Conversion15/1
  Robot/34(S3_AD_Ch2) -> S3ch2_ForceCalibrate/1(In)
  Motor1RatedCurrent/1 -> M1_Current->TorqueCommand/2(RatedCurrent)
  Data Type Conversion17/1 -> Sensor1IMUq3/1  "Sensor1IMUq3"
  Data Type Conversion28/1 -> Sensor3IMUq2/1  "Sensor3IMUq2"
  Robot/22(S1_AD_Ch2) -> S1ch2_ForceCalibrate/1(In)
  Enable/1 -> Robot/Enable
  Robot/26(S1_Quaternions_q3) -> Data Type Conversion17/1
  Robot/31(S2_Quaternions_q2) -> Data Type Conversion22/1
  Robot/28(S2_AD_Ch2) -> Data Type Conversion19/1
  Robot/25(S1_Quaternions_q2) -> Data Type Conversion16/1
  M4_Cnt->Deg/1(Motor1ActuralVelocity) -> Motor2ActuralVelocity/1  "Motor2ActuralVelocity"
  Data Type Conversion16/1 -> Sensor1IMUq2/1  "Sensor1IMUq2"
  Robot/23(S1_Quaternions_q0) -> Data Type Conversion14/1
  Robot/19(M4_DCLinkCircuitVoltage) -> Data Type Conversion11/1
  Robot/37(S3_Quaternions_q2) -> Data Type Conversion28/1
  Robot/38(S3_Quaternions_q3) -> Data Type Conversion29/1
  S3ch1_ForceCalibrate/1(Out) -> Sensor3ADCh1/1  "Sensor3ADCh1"
  Robot/32(S2_Quaternions_q3) -> Data Type Conversion23/1
  Robot/29(S2_Quaternions_q0) -> Data Type Conversion20/1
  Data Type Conversion20/1 -> Sensor2IMUq0/1  "Sensor2IMUq0"
  Robot/33(S3_AD_Ch1) -> S3ch1_ForceCalibrate/1(In)
  S3ch2_ForceCalibrate/1(Out) -> Sensor3ADCh2/1  "Sensor3ADCh2"
  Data Type Conversion14/1 -> Sensor1IMUq0/1  "Sensor1IMUq0"
  Robot/30(S2_Quaternions_q1) -> Data Type Conversion21/1
  Robot/14(M3_DCLinkCircuitVoltage) -> Data Type Conversion8/1
  Data Type Conversion8/1 -> Motor1DCLinkCircuitVoltage/1  "Motor1DCLinkCircuitVoltage"
  S1ch2_ForceCalibrate/1(Out) -> Sensor1ADCh2/1  "Sensor1ADCh2"
  Data Type Conversion21/1 -> Sensor2IMUq1/1  "Sensor2IMUq1"
  Data Type Conversion15/1 -> Sensor1IMUq1/1  "Sensor1IMUq1"
  <Motor1Torque>/1 -> M1_Current->TorqueCommand/1(Current)
  Data Type Conversion18/1 -> Sensor2ADCh1/1  "Sensor2ADCh1"
  Data Type Conversion29/1 -> Sensor3IMUq3/1  "Sensor3IMUq3"
  Data Type Conversion27/1 -> Sensor3IMUq1/1  "Sensor3IMUq1"
  Data Type Conversion22/1 -> Sensor2IMUq2/1  "Sensor2IMUq2"
  <Motor2Torque>/1 -> M2_Current->TorqueCommand/1(Current)
  M2_Current->TorqueCommand/1(Command) -> Robot/2(M2_DesireTorque)
  Motor3RatedCurrent/1 -> M3_Command->Current/1(RatedCurrent), M3_Current->TorqueCommand/2(RatedCurrent)
  Motor4RatedCurrent/1 -> M4_Command->Current/1(RatedCurrent), M24_Current->TorqueCommand/2(RatedCurrent)
  M3_Current->TorqueCommand/1(Command) -> Robot/3(M3_DesireTorque)
  M24_Current->TorqueCommand/1(Command) -> Robot/4(M4_DesireTorque)
  Robot/13(M3_ActuralTorque) -> M3_Command->Current/2(Command)
  M3_Command->Current/1(Current) -> Motor1ActuralTorque/1  "Motor1ActuralTorque"
  M3_PositionCalibrate/1(Motor1ActuralPosition) -> Motor1ActuralPosition/1  "Motor1ActuralPosition"
  Robot/11(M3_ActuralPosition) -> M3_PositionCalibrate/1(M3_ActuralPosition)
  Robot/12(M3_ActuralVelocity) -> M3_Cnt->Deg/1(M3_ActuralVelocity)
  M3_Cnt->Deg/1(Motor1ActuralVelocity) -> Motor1ActuralVelocity/1  "Motor1ActuralVelocity"
  Robot/16(M4_ActuralPosition) -> M4_PositionCalibrate/1(M4_ActuralPosition)
  M4_PositionCalibrate/1(Motor2ActuralPosition) -> Motor2ActuralPosition/1  "Motor2ActuralPosition"
  Robot/17(M4_ActuralVelocity) -> M4_Cnt->Deg/1(M3_ActuralVelocity)
  Motor2RatedCurrent/1 -> M2_Current->TorqueCommand/2(RatedCurrent)
  Robot/18(M4_ActuralTorque) -> M4_Command->Current/2(Command)
  M4_Command->Current/1(Current) -> Motor2ActuralTorque/1  "Motor2ActuralTorque"
  Robot/21(S1_AD_Ch1) -> S1ch1_ForceCalibrate/1(In)
  S1ch1_ForceCalibrate/1(Out) -> Sensor1ADCh1/1  "Sensor1ADCh1"
  <Motor4Torque>/1 -> M24_Current->TorqueCommand/1(Current)
  <Motor3Torque>/1 -> M3_Current->TorqueCommand/1(Current)

== system Robot/Motor1 Torque Control Init Frame/Get MasterState OP Frame ==
  FinishIndex : Inport
  Enable : EnablePort
  Clock : Clock
  Constant4 : Constant  Value=0  OutDataTypeStr=double
  Constant5 : Constant
  Display{1,3..5} (4 alike) : Display
  EtherCAT PDO Receive1 : slrealtimeethercatlib/EtherCAT PDO Receive  Priority=2  sig_name=Drive 1 (Elmo Drive ).Inputs.Status word  sig_offset=744  sig_type=uint16  type_size=16  sig_dim=1  device_id=0  sample_time=0.001000
  Get Device State : slrealtimeethercatlib/Get Device State  device_id=0  slave_name=Drive 1 (Elmo Drive )  sample_time=0.001  slave_addr=1001  selected_slave=Term 1 (EK1100)  timeout=500  slave_found=1
  If Action Subsystem5 : Subsystem  TreatAsAtomicUnit=on
  If Action Subsystem6 : Subsystem  TreatAsAtomicUnit=on
  If Action Subsystem7 : Subsystem  TreatAsAtomicUnit=on
  If1 : If  IfExpression=(u1 == 4663)
  If2 : If  IfExpression=(u1 == 8)
  Merge1 : Merge
  TaskFinished : Outport
  wires:
  If Action Subsystem6/1(Out1) -> Merge1/2
  EtherCAT PDO Receive1/1 -> Display3/1
  Get Device State/1 -> If2/1, Display1/1
  If Action Subsystem7/1(Out1) -> Display5/1
  If Action Subsystem5/1(Out1) -> Merge1/1
  Constant4/1 -> If Action Subsystem6/1(In1)
  If1/1 -> If Action Subsystem7/Action
  Constant5/1 -> If Action Subsystem7/1(In1)
  If2/1 -> If Action Subsystem5/Action
  If2/2 -> If Action Subsystem6/Action
  Clock/1 -> Display4/1
  FinishIndex/1 -> If Action Subsystem5/1(In1)
  Merge1/1 -> TaskFinished/1

== system Robot/Motor1 Torque Control Init Frame/PDO Set 0x6040:6->7->15 Frame ==
  FinishIndex : Inport
  Enable : EnablePort
  Clock : Clock
  Constant : Constant  Value=6  OutDataTypeStr=uint16
  Constant1 : Constant  Value=7  OutDataTypeStr=uint16
  Constant2 : Constant  Value=15  OutDataTypeStr=uint16
  Constant4 : Constant  Value=0  OutDataTypeStr=double
  Constant5 : Constant
  Counter Limited : simulink/Sources/Counter Limited  uplimit=500  tsamp=-1
  Display{1..5} (5 alike) : Display
  EtherCAT PDO Receive1 : slrealtimeethercatlib/EtherCAT PDO Receive  Priority=2  sig_name=Drive 1 (Elmo Drive ).Inputs.Status word  sig_offset=744  sig_type=uint16  type_size=16  sig_dim=1  device_id=0  sample_time=0.001000
  EtherCAT PDO Transmit1 : slrealtimeethercatlib/EtherCAT PDO Transmit  Priority=3  sig_name=Drive 1 (Elmo Drive ).Outputs.Control word  sig_offset=712  sig_type=uint16  type_size=16  sig_dim=1  device_id=0  sample_time=0.001000
  If : If  NumInputs=2  IfExpression=(u1 == 720)&(u2 == 500)  ElseIfExpressions=(u1 == 689)&(u2 == 500), (u1 == 691)&(u2 == 500)
  If Action Subsystem : Subsystem  TreatAsAtomicUnit=on
  If Action Subsystem1 : Subsystem  TreatAsAtomicUnit=on
  If Action Subsystem2 : Subsystem  TreatAsAtomicUnit=on
  If Action Subsystem4 : Subsystem  TreatAsAtomicUnit=on
  If Action Subsystem5 : Subsystem  TreatAsAtomicUnit=on
  If Action Subsystem6 : Subsystem  TreatAsAtomicUnit=on
  If Action Subsystem7 : Subsystem  TreatAsAtomicUnit=on
  If1 : If  IfExpression=(u1 == 4663)|(u1 == 4791)
  If2 : If  IfExpression=(u1 >= 0.1)
  Memory : Memory
  Merge : Merge  Inputs=4
  Merge1 : Merge
  TaskFinished : Outport
  wires:
  If Action Subsystem2/1(Out1) -> Merge/3
  If Action Subsystem7/1(Out1) -> If2/1, Display5/1
  If Action Subsystem6/1(Out1) -> Merge1/2
  EtherCAT PDO Receive1/1 -> If1/1, If/1, Display1/1
  If/2 -> If Action Subsystem1/Action
  Memory/1 -> If Action Subsystem4/1(In1)
  Constant5/1 -> If Action Subsystem7/1(In1)
  Constant1/1 -> If Action Subsystem1/1(In1)
  Constant/1 -> If Action Subsystem/1(In1)
  If Action Subsystem1/1(Out1) -> Merge/2
  If/4 -> If Action Subsystem4/Action
  Constant2/1 -> If Action Subsystem2/1(In1)
  If/3 -> If Action Subsystem2/Action
  If/1 -> If Action Subsystem/Action
  Clock/1 -> Display4/1
  If1/1 -> If Action Subsystem7/Action
  If2/1 -> If Action Subsystem5/Action
  Merge/1 -> Display2/1, EtherCAT PDO Transmit1/1, Memory/1
  FinishIndex/1 -> If Action Subsystem5/1(In1)
  If2/2 -> If Action Subsystem6/Action
  If Action Subsystem4/1(Out1) -> Merge/4
  Counter Limited/1 -> If/2, Display3/1
  Constant4/1 -> If Action Subsystem6/1(In1)
  If Action Subsystem5/1(Out1) -> Merge1/1
  If Action Subsystem/1(Out1) -> Merge/1
  Merge1/1 -> TaskFinished/1

== system Robot/Motor1 Torque Control Init Frame/SDO Get 0x6075 Frame ==
  FinishIndex : Inport
  Enable : EnablePort
  Clock : Clock
  Constant : Constant  OutDataTypeStr=int32
  Constant4 : Constant  Value=0  OutDataTypeStr=double
  Constant5 : Constant
  Display{,1,3..5} (5 alike) : Display
  EtherCAT Async SDO Upload : slrealtimeethercatlib/EtherCAT Async SDO Upload  index=0x6075  subIndex=0  sig_type=uint32  sig_dim=1  device_id=0  slave_name=Drive 1 (Elmo Drive )  sample_time=-1  slave_addr=1001  selected_slave=Term 1 (EK1100)  timeout=3000  slave_found=1  complete=0
  If Action Subsystem5 : Subsystem  TreatAsAtomicUnit=on
  If Action Subsystem6 : Subsystem  TreatAsAtomicUnit=on
  If Action Subsystem7 : Subsystem  TreatAsAtomicUnit=on
  If1 : If  IfExpression=(u1 == 4663)
  If2 : If  IfExpression=(u1 == 2)
  Merge1 : Merge
  TaskFinished : Outport
  RatedCurrent : Outport  Port=2
  wires:
  EtherCAT Async SDO Upload/1 -> RatedCurrent/1, Display/1
  EtherCAT Async SDO Upload/3 -> Display3/1
  EtherCAT Async SDO Upload/2 -> If2/1, Display1/1
  Constant/1 -> EtherCAT Async SDO Upload/1
  If2/1 -> If Action Subsystem5/Action
  Clock/1 -> Display4/1
  If2/2 -> If Action Subsystem6/Action
  If Action Subsystem7/1(Out1) -> Display5/1
  Constant4/1 -> If Action Subsystem6/1(In1)
  If1/1 -> If Action Subsystem7/Action
  If Action Subsystem5/1(Out1) -> Merge1/1
  If Action Subsystem6/1(Out1) -> Merge1/2
  Constant5/1 -> If Action Subsystem7/1(In1)
  FinishIndex/1 -> If Action Subsystem5/1(In1)
  Merge1/1 -> TaskFinished/1

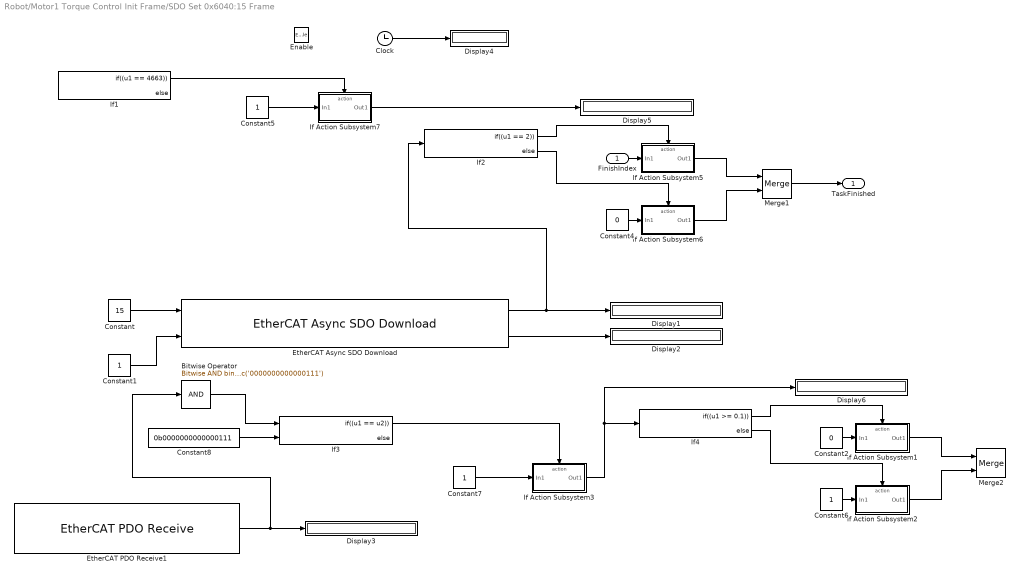
== system Robot/Motor1 Torque Control Init Frame/SDO Set 0x6040:15 Frame ==
  FinishIndex : Inport
  Enable : EnablePort
  Bitwise Operator : simulink/Logic and Bit Operations/Bitwise Operator  logicop=AND  UseBitMask=on  BitMask=bin2dec('0000000000000111')  BitMaskRealWorld=Stored Integer
  Clock : Clock
  Constant : Constant  Value=15  OutDataTypeStr=uint16
  Constant1 : Constant  OutDataTypeStr=int32
  Constant2 : Constant  Value=0  OutDataTypeStr=int32
  Constant4 : Constant  Value=0  OutDataTypeStr=double
  Constant5 : Constant
  Constant6 : Constant  OutDataTypeStr=int32
  Constant7 : Constant
  Constant8 : Constant  Value=0b0000000000000111  OutDataTypeStr=uint16
  Display{1..6} (6 alike) : Display
  EtherCAT Async SDO Download : slrealtimeethercatlib/EtherCAT Async SDO Download  index=0x6040  subIndex=0  sig_type=uint16  sig_dim=1  device_id=0  slave_name=Drive 1 (Elmo Drive )  sample_time=-1  slave_addr=1001  selected_slave=Term 1 (EK1100)  timeout=2000  slave_found=1  complete=0
  EtherCAT PDO Receive1 : slrealtimeethercatlib/EtherCAT PDO Receive  Priority=2  sig_name=Drive 1 (Elmo Drive ).Inputs.Status word  sig_offset=744  sig_type=uint16  type_size=16  sig_dim=1  device_id=0  sample_time=0.001000
  If Action Subsystem1 : Subsystem  TreatAsAtomicUnit=on
  If Action Subsystem2 : Subsystem  TreatAsAtomicUnit=on
  If Action Subsystem3 : Subsystem  TreatAsAtomicUnit=on
  If Action Subsystem5 : Subsystem  TreatAsAtomicUnit=on
  If Action Subsystem6 : Subsystem  TreatAsAtomicUnit=on
  If Action Subsystem7 : Subsystem  TreatAsAtomicUnit=on
  If1 : If  IfExpression=(u1 == 4663)
  If2 : If  IfExpression=(u1 == 2)
  If3 : If  NumInputs=2  IfExpression=(u1 == u2)
  If4 : If  IfExpression=(u1 >= 0.1)
  Merge1 : Merge
  Merge2 : Merge
  TaskFinished : Outport
  wires:
  Constant8/1 -> If3/2
  Bitwise Operator/1 -> If3/1
  If Action Subsystem3/1(Out1) -> Display6/1, If4/1
  Clock/1 -> Display4/1
  If Action Subsystem2/1(Out1) -> Merge2/2
  If Action Subsystem1/1(Out1) -> Merge2/1
  Constant7/1 -> If Action Subsystem3/1(In1)
  If2/2 -> If Action Subsystem6/Action
  EtherCAT PDO Receive1/1 -> Display3/1, Bitwise Operator/1
  If3/1 -> If Action Subsystem3/Action
  If4/1 -> If Action Subsystem1/Action
  Constant6/1 -> If Action Subsystem2/1(In1)
  If4/2 -> If Action Subsystem2/Action
  EtherCAT Async SDO Download/1 -> If2/1, Display1/1
  Constant4/1 -> If Action Subsystem6/1(In1)
  Constant5/1 -> If Action Subsystem7/1(In1)
  Constant1/1 -> EtherCAT Async SDO Download/2
  If Action Subsystem6/1(Out1) -> Merge1/2
  If Action Subsystem7/1(Out1) -> Display5/1
  If2/1 -> If Action Subsystem5/Action
  Constant2/1 -> If Action Subsystem1/1(In1)
  If1/1 -> If Action Subsystem7/Action
  FinishIndex/1 -> If Action Subsystem5/1(In1)
  EtherCAT Async SDO Download/2 -> Display2/1
  Constant/1 -> EtherCAT Async SDO Download/1
  If Action Subsystem5/1(Out1) -> Merge1/1
  Merge1/1 -> TaskFinished/1

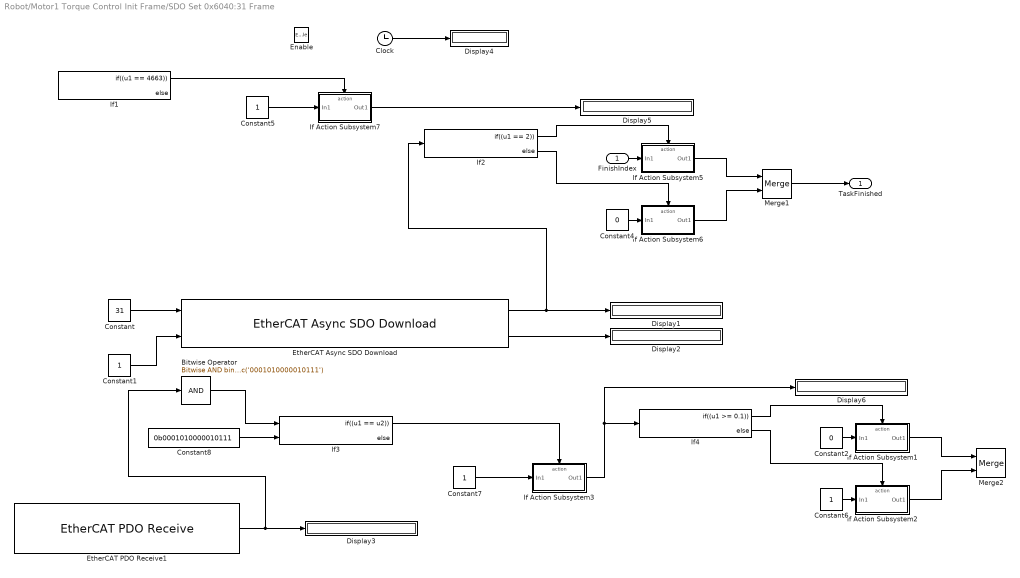
== system Robot/Motor1 Torque Control Init Frame/SDO Set 0x6040:31 Frame ==
  FinishIndex : Inport
  Enable : EnablePort
  Bitwise Operator : simulink/Logic and Bit Operations/Bitwise Operator  logicop=AND  UseBitMask=on  BitMask=bin2dec('0001010000010111')  BitMaskRealWorld=Stored Integer
  Clock : Clock
  Constant : Constant  Value=31  OutDataTypeStr=uint16
  Constant1 : Constant  OutDataTypeStr=int32
  Constant2 : Constant  Value=0  OutDataTypeStr=int32
  Constant4 : Constant  Value=0  OutDataTypeStr=double
  Constant5 : Constant
  Constant6 : Constant  OutDataTypeStr=int32
  Constant7 : Constant
  Constant8 : Constant  Value=0b0001010000010111  OutDataTypeStr=uint16
  Display{1..6} (6 alike) : Display
  EtherCAT Async SDO Download : slrealtimeethercatlib/EtherCAT Async SDO Download  index=0x6040  subIndex=0  sig_type=uint16  sig_dim=1  device_id=0  slave_name=Drive 1 (Elmo Drive )  sample_time=-1  slave_addr=1001  selected_slave=Term 1 (EK1100)  timeout=2000  slave_found=1  complete=0
  EtherCAT PDO Receive1 : slrealtimeethercatlib/EtherCAT PDO Receive  Priority=2  sig_name=Drive 1 (Elmo Drive ).Inputs.Status word  sig_offset=744  sig_type=uint16  type_size=16  sig_dim=1  device_id=0  sample_time=0.001000
  If Action Subsystem1 : Subsystem  TreatAsAtomicUnit=on
  If Action Subsystem2 : Subsystem  TreatAsAtomicUnit=on
  If Action Subsystem3 : Subsystem  TreatAsAtomicUnit=on
  If Action Subsystem5 : Subsystem  TreatAsAtomicUnit=on
  If Action Subsystem6 : Subsystem  TreatAsAtomicUnit=on
  If Action Subsystem7 : Subsystem  TreatAsAtomicUnit=on
  If1 : If  IfExpression=(u1 == 4663)
  If2 : If  IfExpression=(u1 == 2)
  If3 : If  NumInputs=2  IfExpression=(u1 == u2)
  If4 : If  IfExpression=(u1 >= 0.1)
  Merge1 : Merge
  Merge2 : Merge
  TaskFinished : Outport
  wires:
  If1/1 -> If Action Subsystem7/Action
  If Action Subsystem5/1(Out1) -> Merge1/1
  If Action Subsystem6/1(Out1) -> Merge1/2
  FinishIndex/1 -> If Action Subsystem5/1(In1)
  If2/1 -> If Action Subsystem5/Action
  If4/2 -> If Action Subsystem2/Action
  EtherCAT Async SDO Download/1 -> If2/1, Display1/1
  Constant/1 -> EtherCAT Async SDO Download/1
  Bitwise Operator/1 -> If3/1
  If Action Subsystem7/1(Out1) -> Display5/1
  Constant8/1 -> If3/2
  If2/2 -> If Action Subsystem6/Action
  If Action Subsystem3/1(Out1) -> Display6/1, If4/1
  If Action Subsystem2/1(Out1) -> Merge2/2
  If3/1 -> If Action Subsystem3/Action
  Constant4/1 -> If Action Subsystem6/1(In1)
  Constant6/1 -> If Action Subsystem2/1(In1)
  If4/1 -> If Action Subsystem1/Action
  Constant1/1 -> EtherCAT Async SDO Download/2
  EtherCAT PDO Receive1/1 -> Display3/1, Bitwise Operator/1
  Clock/1 -> Display4/1
  If Action Subsystem1/1(Out1) -> Merge2/1
  Constant2/1 -> If Action Subsystem1/1(In1)
  EtherCAT Async SDO Download/2 -> Display2/1
  Constant5/1 -> If Action Subsystem7/1(In1)
  Constant7/1 -> If Action Subsystem3/1(In1)
  Merge1/1 -> TaskFinished/1
